simulink model "Opcode_Decoder"  (R2024b)
settings: Solver=VariableStepAuto  StartTime=0.0  StopTime=10.0  RelTol=1e-3
settings Model: Creator=HP  LastModifiedBy=HP

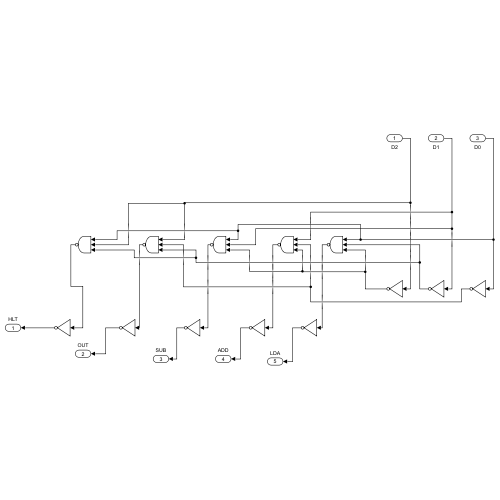
[thumbnail: Simulink's stored preview of the top-level diagram]
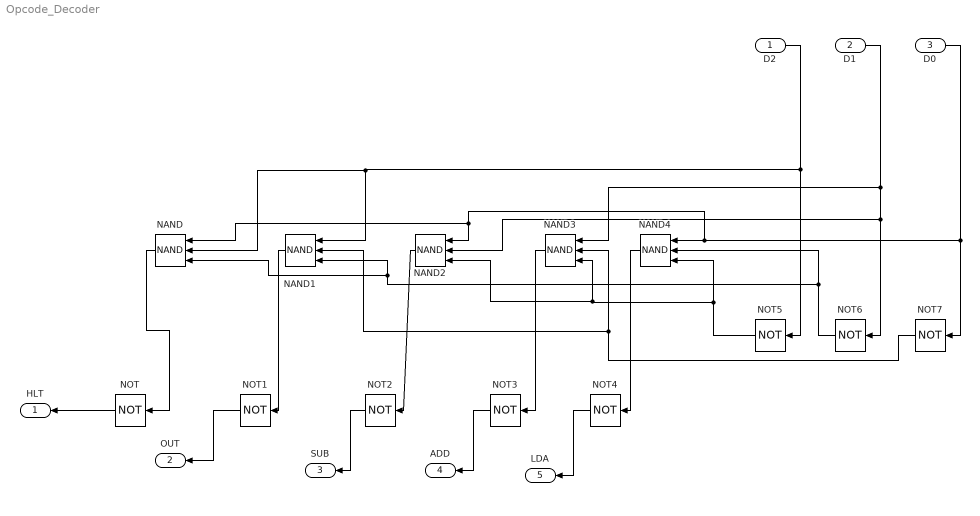
== system Opcode_Decoder ==
  D2 : Inport
  D1 : Inport  Port=2
  D0 : Inport  Port=3
  NAND{,1..4} (5 alike) : Logic  Operator=NAND  Inputs=3  IconShape=distinctive  AllPortsSameDT=off  OutDataTypeStr=boolean
  NOT{,1..7} (8 alike) : Logic  Operator=NOT  IconShape=distinctive  AllPortsSameDT=off  OutDataTypeStr=boolean
  HLT : Outport
  OUT : Outport  Port=2
  SUB : Outport  Port=3
  ADD : Outport  Port=4
  LDA : Outport  Port=5
  wires:
  D2/1 -> NAND/2, NAND1/1, NOT5/1
  D0/1 -> NAND/1, NAND2/1, NAND4/1, NOT7/1
  NOT5/1 -> NAND2/3, NAND3/3, NAND4/3
  NOT6/1 -> NAND/3, NAND1/3, NAND4/2
  D1/1 -> NAND3/1, NAND2/2, NOT6/1
  NOT7/1 -> NAND1/2, NAND3/2
  NAND4/1 -> NOT4/1
  NAND3/1 -> NOT3/1
  NAND2/1 -> NOT2/1
  NAND1/1 -> NOT1/1
  NAND/1 -> NOT/1
  NOT/1 -> HLT/1
  NOT1/1 -> OUT/1
  NOT2/1 -> SUB/1
  NOT3/1 -> ADD/1
  NOT4/1 -> LDA/1
